simulink model "PID_lab4"  (R2019b)
settings: Solver=VariableStepAuto  StartTime=0.0  StopTime=10.0  RelTol=1e-3
values from neighbouring files (symbols this model uses):
  angle_1 = 3.14    [lab4.m]
  J = 0.0023    [lab4.m]
  Kb = 5    [lab4.m]
  Kd = 0.03    [lab4.m]
  Ke = Km    (= 0.29)    [lab4.m]
  Ki = 0.05    [lab4.m]
  Km = 0.29    [lab4.m]
  Kp = 3    [lab4.m]
  L = 0.0047    [lab4.m]
  R = 4.7    [lab4.m]
  Um = 3.5    [lab4.m]
libraries: simulink x1
settings Model: Creator=Ivan  LastModifiedBy=Ivan

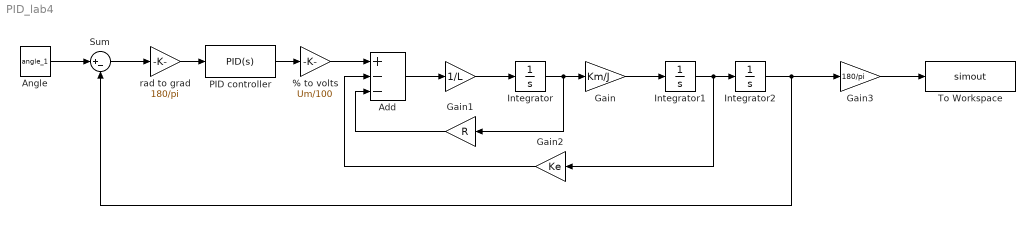
== system PID_lab4 ==
  " " : Gain  Gain=1/L
  % to volts : Gain  Gain=Um/100
  Add : Sum  Inputs=+--
  Angle : Constant  Value=angle_1  VectorParams1D=off
  Gain : Gain  Gain=Km/J
  Gain1 : Gain  Gain=R
  Gain2 : Gain  Gain=Ke
  Gain3 : Gain  Gain=180/pi
  Integrator : Integrator
  Integrator1 : Integrator
  Integrator2 : Integrator
  PID controller : simulink/Continuous/PID Controller  Controller=PID  Form=Parallel  TimeDomain=Continuous-time  SampleTime=-1  IntegratorMethod=Forward Euler  FilterMethod=Forward Euler  ControllerParametersSource=internal  P=Kp  I=Ki  D=Kd  UseFilter=on  N=0  TunerSelectOption=Transfer Function Based (PID Tuner App)  InitialConditionSource=internal  InitialConditionForIntegrator=0  InitialConditionForFilter=0  DifferentiatorICPrevScaledInput=0  ExternalReset=none  TrackingMode=off  Kt=1  LimitOutput=on  UpperSaturationLimit=100  LowerSaturationLimit=-100  LinearizeAsGain=off  AntiWindupMode=back-calculation  Kb=Kb  POutMin=[]  POutMax=[]  IOutMin=[]  IOutMax=[]  DOutMin=[]  DOutMax=[]  NOutMin=[]  NOutMax=[]  SumOutMin=[]  SumOutMax=[]  SaturationOutMin=[]  SaturationOutMax=[]  PParamMin=[]  PParamMax=[]  IParamMin=[]  IParamMax=[]  DParamMin=[]  DParamMax=[]  NParamMin=[]  NParamMax=[]  KbParamMin=[]  KbParamMax=[]  KtParamMin=[]  KtParamMax=[]  KbOutMin=[]  KbOutMax=[]  KtOutMin=[]  KtOutMax=[]  IntegratorOutMin=[]  IntegratorOutMax=[]  FilterOutMin=[]  FilterOutMax=[]  SumI1OutMin=[]  SumI1OutMax=[]  SumI2OutMin=[]  SumI2OutMax=[]  SumI3OutMin=[]  SumI3OutMax=[]  SumI4OutMin=[]  SumI4OutMax=[]  SumDOutMin=[]  SumDOutMax=[]  DifferentiatorOutMin=[]  DifferentiatorOutMax=[]  FilterDiffOutCoefMin=[]  FilterDiffOutCoefMax=[]  ReciprocalOutMin=[]  ReciprocalOutMax=[]  SumDenOutMin=[]  SumDenOutMax=[]  SumNumOutMin=[]  SumNumOutMax=[]  DivideOutMin=[]  DivideOutMax=[]  IntegratorContinuousStateAttributes=''  IntegratorStateMustResolveToSignalObject=off  IntegratorRTWStateStorageClass=Auto  FilterContinuousStateAttributes=''  FilterStateMustResolveToSignalObject=off  FilterRTWStateStorageClass=Auto  ParallelPVariant=InternalParameters  IdealPVariant=Disabled  IVariant=InternalParameters  DVariant=InternalParameters  IntegratorVariant=Continuous  SatVariant=Enabled  AWVariant=BackCalculation  PCopyVariant=Disabled  TRVariant=Disabled  FdbkBlocksVariant=Forward  IdealPFdbkVariant=Disabled  SatFdbkVariant=Disabled  DerivativeFilterVariant=ContFilter  NVariant=InternalParameters  NCopyVariant=Disabled  FilterICVariant=InternalICsFilter  IntegratorICVariant=InternalICs  ExternalResetVariant=Disabled  TRSumVariant=Passthrough  SumFdbkVariant=Disabled  SumVariant=Sum_PID
  Sum : Sum  Inputs=|+-
  To Workspace : ToWorkspace  VariableName=simout  SaveFormat=Timeseries  SampleTime=-1
  rad to grad : Gain  Gain=180/pi
  wires:
  Angle/1 -> Sum/1
  rad to grad/1 -> PID controller/1
  Sum/1 -> rad to grad/1
  PID controller/1 -> % to volts/1
  % to volts/1 -> Add/1
  Add/1 -> " "/1
  " "/1 -> Integrator/1
  Integrator/1 -> Gain1/1, Gain/1
  Gain1/1 -> Add/3
  Gain/1 -> Integrator1/1
  Integrator1/1 -> Gain2/1, Integrator2/1
  Gain2/1 -> Add/2
  Integrator2/1 -> Gain3/1, Sum/2
  Gain3/1 -> To Workspace/1
